simulink model "electrical_model"  (R2016a)
settings: Solver=FixedStepAuto  StartTime=0.0  StopTime=3  FixedStep=Ts  RelTol=1e-3
values from neighbouring files (symbols this model uses):
  Li = 0.16e-3    (= 0.00016)    [Model.m]
  ri = 0.1    [Model.m]
  Ts = 1    [MPC.m]    (also in Model.m = 0.0001)
  w_g = N*pi/30    (= 2.35619449019)    [Model.m]
undefined symbols (not defined in the file or in its folder): Continuous, DiscIntNeverNeededParam, spsPMSynchronousMachineModel
libraries: dspsrcs4 x3, powerlib x1
settings Model: Creator=syf  LastModifiedBy=syf
settings SolverCC: AutoInsertRateTranBlk=on

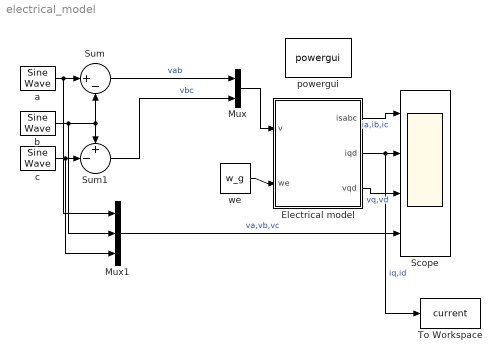
== system electrical_model ==
  Electrical model : Subsystem  AncestorBlock=spsPMSynchronousMachineModel/Continuous
  Mux : Mux  Inputs=2
  Mux1 : Mux  Inputs=3
  Scope : Scope  NumInputPorts=4
  Sum : Sum  Inputs=|+-
  Sum1 : Sum  Inputs=+-|
  To Workspace : ToWorkspace  VariableName=current  SampleTime=-1
  a : dspsrcs4/Sine Wave  Amplitude=200  Frequency=w_g/(2*pi)  Phase=0  SampleMode=Discrete  OutComplex=Real  CompMethod=Trigonometric fcn  TableSize=Speed  SampleTime=Ts  SamplesPerFrame=1  ResetState=Restart at time zero  OutputFrames=off  dataType=double  wordLen=16  udDataType=sfix(16)  fracBitsMode=Best precision  numFracBits=15  OutDataTypeStr=double  LastOutDataTypeStr=double
  b : dspsrcs4/Sine Wave  Amplitude=200  Frequency=w_g/(2*pi)  Phase=2*pi/3  SampleMode=Discrete  OutComplex=Real  CompMethod=Trigonometric fcn  TableSize=Speed  SampleTime=Ts  SamplesPerFrame=1  ResetState=Restart at time zero  OutputFrames=off  dataType=double  wordLen=16  udDataType=sfix(16)  fracBitsMode=Best precision  numFracBits=15  OutDataTypeStr=double  LastOutDataTypeStr=double
  c : dspsrcs4/Sine Wave  Amplitude=200  Frequency=w_g/(2*pi)  Phase=-2*pi/3  SampleMode=Discrete  OutComplex=Real  CompMethod=Trigonometric fcn  TableSize=Speed  SampleTime=Ts  SamplesPerFrame=1  ResetState=Restart at time zero  OutputFrames=off  dataType=double  wordLen=16  udDataType=sfix(16)  fracBitsMode=Best precision  numFracBits=15  OutDataTypeStr=double  LastOutDataTypeStr=double
  powergui : powerlib/powergui  Priority=1  SimulationMode=Discrete  SolverType=Backward Euler  SampleTime=Ts  frequency=60  SPID=off  DisableSnubberDevices=off  DisableRonSwitches=off  DisableVfSwitches=off  SwTol=0  DisplayEquations=off  Interpol=off  ExternalGateDelay=off  methode=off  Ts=10  FunctionMessages=off  echomessages=off  HookPort=off  EnableUseOfTLC=off  x0status=blocks  frequencyindice=60  Pbase=100e6  ErrMax=1e-4  Iterations=50  UnitsV=kV  UnitsW=MW  buscounter=0  RestoreLinks=warning  ResistiveCurrentMeasurement=off  Frange=[0:2:500]  Ylog=off  Xlog=on  ShowGrid=off  save=off  variable=ZData  structure=0  ZoomFFT=off  StartTime=0.0  cycles=1  DisplayStyle=1  fundamental=60  FreqAxis=off  MaxFrequency=1000  frequencyindicesteady=1  RmsSteady=1  display=off
  we : Constant  Value=w_g
  wires:
  we/1 -> Electrical model/2(we)
  Mux/1 -> Electrical model/1(v)
  Sum/1 -> Mux/1  "vab"
  Sum1/1 -> Mux/2  "vbc"
  Electrical model/1(isabc) -> Scope/1  "ia,ib,ic"
  Electrical model/2(iqd) -> To Workspace/1, Scope/2  "iq,id"
  Electrical model/3(vqd) -> Scope/3  "vq,vd"
  a/1 -> Mux1/1, Sum/1
  b/1 -> Mux1/2, Sum1/1, Sum/2
  c/1 -> Mux1/3, Sum1/2
  Mux1/1 -> Scope/4  "va,vb,vc"

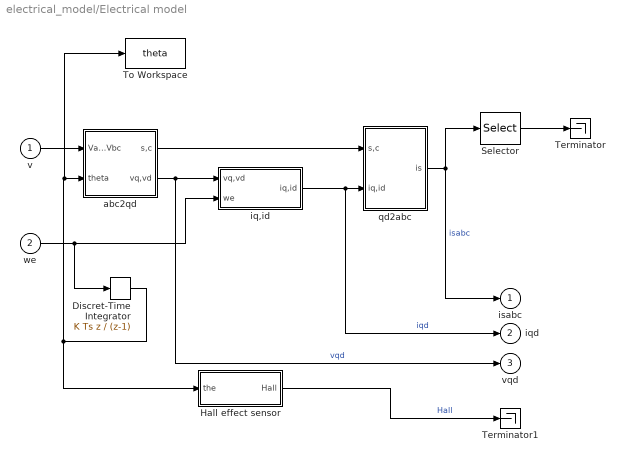
== system electrical_model/Electrical model ==
  v : Inport
  we : Inport  Port=2
  Discret-Time Integrator : DiscreteIntegrator  IntegratorMethod=Integration: Backward Euler  gainval=1  InitialConditionSetting=State (most efficient)  SampleTime=Ts  ICPrevOutput=DiscIntNeverNeededParam  ICPrevScaledInput=DiscIntNeverNeededParam
  Hall effect sensor : Subsystem
  Selector : Selector  InputPortWidth=3  IndexOptions=Index vector (dialog)  Indices=1:2  OutputSizes=1
  Terminator : Terminator
  Terminator1 : Terminator
  To Workspace : ToWorkspace  VariableName=theta  SampleTime=-1
      settings: Save2DSignal=2-D array (concatenate along first dimension)
  abc2qd : Subsystem
  iq,id : Subsystem
  qd2abc : Subsystem
  isabc : Outport  InitialOutput=0
  iqd : Outport  Port=2  InitialOutput=0
  vqd : Outport  Port=3  InitialOutput=0
  wires:
  Hall effect sensor/1(Hall) -> Terminator1/1  "Hall"
  Selector/1 -> Terminator/1
  qd2abc/1(is) -> isabc/1, Selector/1  "isabc"
  iq,id/1(iq,id) -> iqd/1, qd2abc/2(iq,id)  "iqd"
  v/1 -> abc2qd/1(Vab,Vbc)
  abc2qd/1(s,c) -> qd2abc/1(s,c)
  abc2qd/2(vq,vd) -> vqd/1, iq,id/1(vq,vd)  "vqd"
  Discret-Time Integrator/1 -> Hall effect sensor/1(the), To Workspace/1, abc2qd/2(theta)
  we/1 -> iq,id/2(we), Discret-Time Integrator/1

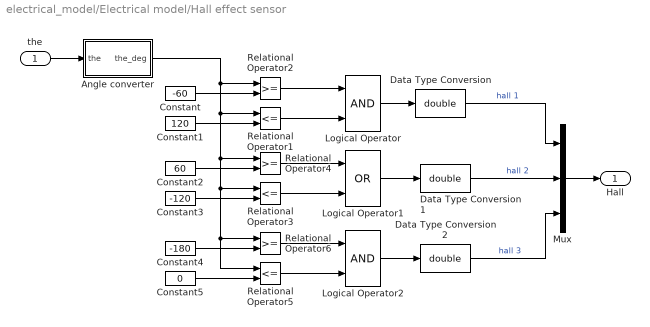
== system electrical_model/Electrical model/Hall effect sensor ==
  the : Inport
  Angle converter : Subsystem
  Constant : Constant  Value=-60
  Constant1 : Constant  Value=120
  Constant2 : Constant  Value=60
  Constant3 : Constant  Value=-120
  Constant4 : Constant  Value=-180
  Constant5 : Constant  Value=0
  Data Type Conversion : DataTypeConversion  OutDataTypeStr=double  SaturateOnIntegerOverflow=on  RndMeth=Zero
  Data Type Conversion1 : DataTypeConversion  OutDataTypeStr=double  SaturateOnIntegerOverflow=on  RndMeth=Zero
  Data Type Conversion2 : DataTypeConversion  OutDataTypeStr=double  SaturateOnIntegerOverflow=on  RndMeth=Zero
  Logical Operator : Logic  AllPortsSameDT=off  OutDataTypeStr=boolean
  Logical Operator1 : Logic  Operator=OR  AllPortsSameDT=off  OutDataTypeStr=boolean
  Logical Operator2 : Logic  AllPortsSameDT=off  OutDataTypeStr=boolean
  Mux : Mux  Inputs=3
  Relational Operator1 : RelationalOperator  Operator=<=  InputSameDT=on
  Relational Operator2 : RelationalOperator  InputSameDT=on
  Relational Operator3 : RelationalOperator  Operator=<=  InputSameDT=on
  Relational Operator4 : RelationalOperator  InputSameDT=on
  Relational Operator5 : RelationalOperator  Operator=<=  InputSameDT=on
  Relational Operator6 : RelationalOperator  InputSameDT=on
  Hall : Outport
  wires:
  Mux/1 -> Hall/1
  Data Type Conversion2/1 -> Mux/3  "hall 3"
  Data Type Conversion1/1 -> Mux/2  "hall 2"
  Data Type Conversion/1 -> Mux/1  "hall 1"
  Relational Operator5/1 -> Logical Operator2/2
  Logical Operator2/1 -> Data Type Conversion2/1
  Relational Operator6/1 -> Logical Operator2/1
  Constant4/1 -> Relational Operator6/2
  Constant5/1 -> Relational Operator5/2
  Relational Operator3/1 -> Logical Operator1/2
  Logical Operator1/1 -> Data Type Conversion1/1
  Logical Operator/1 -> Data Type Conversion/1
  Relational Operator2/1 -> Logical Operator/1
  Relational Operator1/1 -> Logical Operator/2
  Angle converter/1(the_deg) -> Relational Operator2/1, Relational Operator1/1, Relational Operator6/1, Relational Operator5/1, Relational Operator3/1, Relational Operator4/1
  Constant/1 -> Relational Operator2/2
  Constant1/1 -> Relational Operator1/2
  Relational Operator4/1 -> Logical Operator1/1
  Constant2/1 -> Relational Operator4/2
  Constant3/1 -> Relational Operator3/2
  the/1 -> Angle converter/1(the)

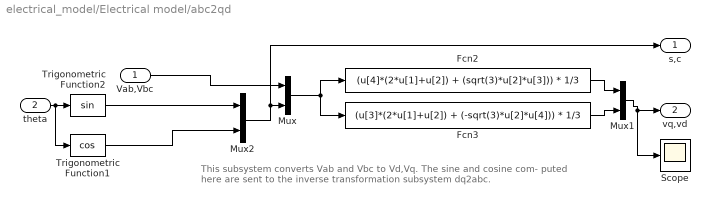
== system electrical_model/Electrical model/abc2qd ==
  note: This subsystem converts Vab and Vbc to Vd,Vq. The sine and cosine com-
      | puted here are sent to the inverse transformation subsystem dq2abc.
  Vab,Vbc : Inport
  theta : Inport  Port=2
  Fcn2 : Fcn  Expr=(u[4]*(2*u[1]+u[2]) + (sqrt(3)*u[2]*u[3])) * 1/3
  Fcn3 : Fcn  Expr=(u[3]*(2*u[1]+u[2]) + (-sqrt(3)*u[2]*u[4])) * 1/3
  Mux : Mux  Inputs=2
  Mux1 : Mux  Inputs=2
  Mux2 : Mux  Inputs=2
  Scope : Scope
  Trigonometric Function1 : Trigonometry  Operator=cos  SampleTime=Ts
  Trigonometric Function2 : Trigonometry  SampleTime=Ts
  s,c : Outport  InitialOutput=0
  vq,vd : Outport  Port=2  InitialOutput=0
  wires:
  Vab,Vbc/1 -> Mux/1
  Mux1/1 -> Scope/1, vq,vd/1
  Fcn2/1 -> Mux1/1
  Mux2/1 -> Mux/2, s,c/1
  Mux/1 -> Fcn3/1, Fcn2/1
  Fcn3/1 -> Mux1/2
  Trigonometric Function2/1 -> Mux2/1
  Trigonometric Function1/1 -> Mux2/2
  theta/1 -> Trigonometric Function1/1, Trigonometric Function2/1

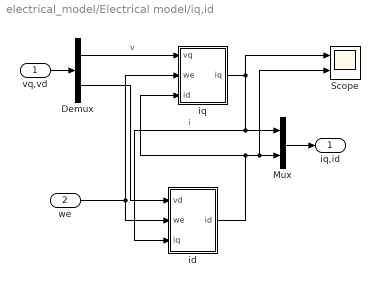
== system electrical_model/Electrical model/iq,id ==
  vq,vd : Inport
  we : Inport  Port=2
  Demux : Demux  Outputs=2
  Mux : Mux  Inputs=2
  Scope : Scope  NumInputPorts=2
  id : Subsystem
  iq : Subsystem
  iq,id : Outport  InitialOutput=0
  wires:
  Mux/1 -> iq,id/1
  vq,vd/1 -> Demux/1
  Demux/1 -> iq/1(vq)  "v"
  Demux/2 -> id/1(vd)
  iq/1(iq) -> Scope/1, id/3(iq), Mux/1  "i"
  we/1 -> id/2(we), iq/2(we)
  id/1(id) -> iq/3(id), Scope/2, Mux/2

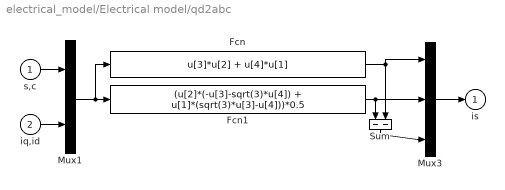
== system electrical_model/Electrical model/qd2abc ==
  s,c : Inport
  iq,id : Inport  Port=2
  Fcn : Fcn  Expr=u[3]*u[2] + u[4]*u[1]
  Fcn1 : Fcn  Expr=(u[2]*(-u[3]-sqrt(3)*u[4]) + u[1]*(sqrt(3)*u[3]-u[4]))*0.5
  Mux1 : Mux  Inputs=2
  Mux3 : Mux  Inputs=3
  Sum : Sum  Inputs=--  SaturateOnIntegerOverflow=on  InputSameDT=on  OutDataTypeStr=Inherit: Same as first input
  is : Outport  InitialOutput=0
  wires:
  Mux3/1 -> is/1
  Fcn1/1 -> Mux3/2, Sum/1
  Fcn/1 -> Mux3/1, Sum/2
  Sum/1 -> Mux3/3
  iq,id/1 -> Mux1/2
  s,c/1 -> Mux1/1
  Mux1/1 -> Fcn1/1, Fcn/1

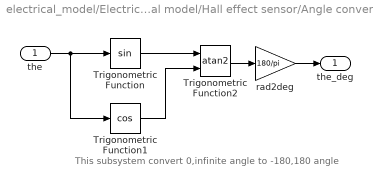
== system electrical_model/Electrical model/Hall effect sensor/Angle converter ==
  note: This subsystem convert 0,infinite angle to -180,180 angle
  the : Inport
  Trigonometric Function : Trigonometry
  Trigonometric Function1 : Trigonometry  Operator=cos
  Trigonometric Function2 : Trigonometry  Operator=atan2
  rad2deg : Gain  Gain=180/pi  SaturateOnIntegerOverflow=on  OutDataTypeStr=Inherit: Same as input  ParamDataTypeStr=Inherit: Same as input
  the_deg : Outport
  wires:
  the/1 -> Trigonometric Function/1, Trigonometric Function1/1
  Trigonometric Function/1 -> Trigonometric Function2/1
  Trigonometric Function1/1 -> Trigonometric Function2/2
  Trigonometric Function2/1 -> rad2deg/1
  rad2deg/1 -> the_deg/1

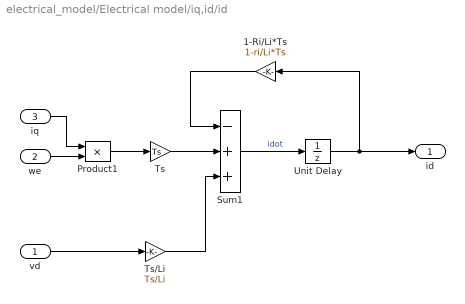
== system electrical_model/Electrical model/iq,id/id ==
  vd : Inport
  we : Inport  Port=2
  iq : Inport  Port=3
  1-Ri/Li*Ts : Gain  Gain=1-ri/Li*Ts  SaturateOnIntegerOverflow=on  OutDataTypeStr=Inherit: Same as input  ParamDataTypeStr=Inherit: Same as input
  Product1 : Product  SaturateOnIntegerOverflow=on  InputSameDT=on  OutDataTypeStr=Inherit: Same as first input
  Sum1 : Sum  Inputs=-++  SaturateOnIntegerOverflow=on  InputSameDT=on  OutDataTypeStr=Inherit: Same as first input
  Ts : Gain  Gain=Ts  SaturateOnIntegerOverflow=on  OutDataTypeStr=Inherit: Same as input  ParamDataTypeStr=Inherit: Same as input
  Ts/Li : Gain  Gain=Ts/Li  SaturateOnIntegerOverflow=on  OutDataTypeStr=Inherit: Same as input  ParamDataTypeStr=Inherit: Same as input
  Unit Delay : UnitDelay  SampleTime=-1
  id : Outport  InitialOutput=0
  wires:
  1-Ri/Li*Ts/1 -> Sum1/1
  Ts/1 -> Sum1/2
  Sum1/1 -> Unit Delay/1  "idot"
  Product1/1 -> Ts/1
  Ts/Li/1 -> Sum1/3
  iq/1 -> Product1/1
  vd/1 -> Ts/Li/1
  we/1 -> Product1/2
  Unit Delay/1 -> id/1, 1-Ri/Li*Ts/1

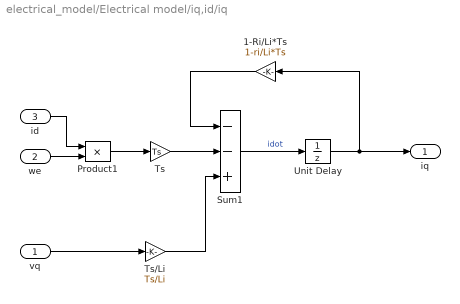
== system electrical_model/Electrical model/iq,id/iq ==
  vq : Inport
  we : Inport  Port=2
  id : Inport  Port=3
  1-Ri/Li*Ts : Gain  Gain=1-ri/Li*Ts  SaturateOnIntegerOverflow=on  OutDataTypeStr=Inherit: Same as input  ParamDataTypeStr=Inherit: Same as input
  Product1 : Product  SaturateOnIntegerOverflow=on  InputSameDT=on  OutDataTypeStr=Inherit: Same as first input
  Sum1 : Sum  Inputs=--+  SaturateOnIntegerOverflow=on  InputSameDT=on  OutDataTypeStr=Inherit: Same as first input
  Ts : Gain  Gain=Ts  SaturateOnIntegerOverflow=on  OutDataTypeStr=Inherit: Same as input  ParamDataTypeStr=Inherit: Same as input
  Ts/Li : Gain  Gain=Ts/Li  SaturateOnIntegerOverflow=on  OutDataTypeStr=Inherit: Same as input  ParamDataTypeStr=Inherit: Same as input
  Unit Delay : UnitDelay  SampleTime=-1
  iq : Outport  InitialOutput=0
  wires:
  1-Ri/Li*Ts/1 -> Sum1/1
  Ts/1 -> Sum1/2
  Sum1/1 -> Unit Delay/1  "idot"
  Product1/1 -> Ts/1
  Ts/Li/1 -> Sum1/3
  id/1 -> Product1/1
  vq/1 -> Ts/Li/1
  we/1 -> Product1/2
  Unit Delay/1 -> 1-Ri/Li*Ts/1, iq/1
